simulink library "INT_PhyMod_OpModeSelect"  (R2016b)
settings: Solver=VariableStepAuto  StartTime=0.0  StopTime=10.0  RelTol=1e-3
settings Model: Creator=Administrator  LastModifiedBy=Administrator

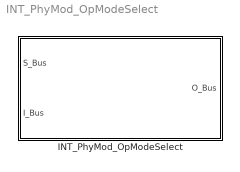
== system INT_PhyMod_OpModeSelect ==
  INT_PhyMod_OpModeSelect : Subsystem

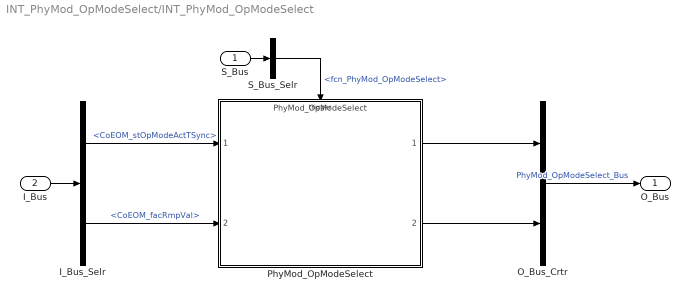
== system INT_PhyMod_OpModeSelect/INT_PhyMod_OpModeSelect ==
  S_Bus : Inport
  I_Bus : Inport  Port=2
  I_Bus_Selr : BusSelector  OutputSignals=CoEOM_stOpModeActTSync,CoEOM_facRmpVal
  O_Bus_Crtr : BusCreator  Inputs=2
  PhyMod_OpModeSelect : ModelReference  ModelNameDialog=PhyMod_OpModeSelect  SimulationMode=Normal  ModelReferenceVersion=1.3  TriggerPortName=function  TriggerPortTriggerType=function-call  TriggerPortStatesWhenEnabling=held
  S_Bus_Selr : BusSelector  OutputSignals=fcn_PhyMod_OpModeSelect
  O_Bus : Outport
  wires:
  S_Bus_Selr/1 -> PhyMod_OpModeSelect/Trigger  "<fcn_PhyMod_OpModeSelect>"
  S_Bus/1 -> S_Bus_Selr/1
  I_Bus/1 -> I_Bus_Selr/1
  I_Bus_Selr/1 -> PhyMod_OpModeSelect/1  "<CoEOM_stOpModeActTSync>"
  I_Bus_Selr/2 -> PhyMod_OpModeSelect/2  "<CoEOM_facRmpVal>"
  O_Bus_Crtr/1 -> O_Bus/1  "PhyMod_OpModeSelect_Bus"
  PhyMod_OpModeSelect/1 -> O_Bus_Crtr/1
  PhyMod_OpModeSelect/2 -> O_Bus_Crtr/2
